simulink model "fullVehicleModel_17b"  (R2017b)
settings: Solver=VariableStepAuto  StartTime=0.0  StopTime=10.0  RelTol=1e-3
undefined symbols (not defined in the file): ambient_temp, bat, bat_r1, Batt, batt_initCharge, Batt_sensorLag_s, bvatt_AhRating, DiscIntNeverNeededParam, electronics_power, env, module_broad_area, module_small_area, module_top_area, mot, no_module, shifterPos, Ts, Ts_elec
libraries: Soft_ECUs x90, fl_lib x67, nesl_utility x29, Battery_lib x28, Gen_lib x13, simulink x10, aerolibconvert2 x7, SoftCAN_Interface x6, autolibshared x2, Additional_blocks_lib x1, elec_lib x1
(part 1 of 4)
settings Model: Creator=carca  LastModifiedBy=Truman

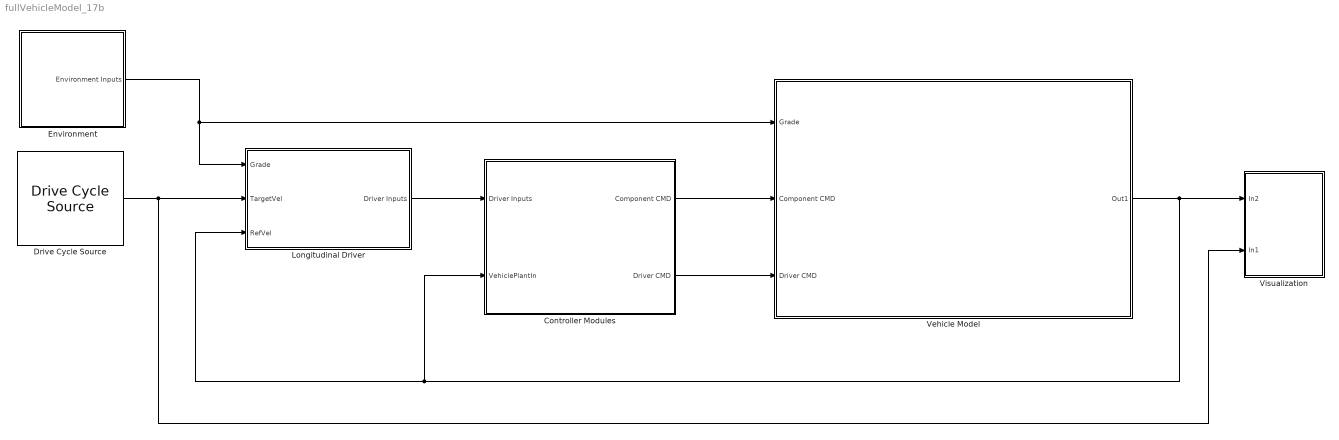
== system fullVehicleModel_17b ==
  "Controller Modules " : Subsystem
      mask Display: image('C:\Users\carca\Desktop\Icon Images\controllerMask.png');
  Drive Cycle Source : autolibshared/Drive Cycle Source  cycleVar=FTP75  fileVar=cycleFTP75.mat  tfinal="2474  seconds"  cycleRepeat=off  outAccPort=off  t_wot1=5  xdot_woto=0  xdot_wot1=30  t_wot2=20  xdot_wot2=0  t_wotend=30  srcUnit=m/s  outUnit=m/s  srcAccUnit=m/s/s  outAccUnit=m/s^2  dt=0
      settings: SourceProductName=Powertrain Blockset  SourceProductBaseCode=PW
  Environment : Subsystem
      mask Display: image('C:\Users\carca\Desktop\Icon Images\environmentMask.png');
  Longitudinal Driver : Subsystem
      mask Display: image('C:\Users\carca\Desktop\Icon Images\driverMask.png');
  Vehicle Model : Subsystem
      mask Display: image('C:\Users\carca\Desktop\Icon Images\camaroMask.png');
  "Visualization " : Subsystem
  wires:
  Environment/1(Environment Inputs) -> Longitudinal Driver/1(Grade), Vehicle Model/1(Grade)
  "Controller Modules "/1(Component CMD) -> Vehicle Model/2(Component CMD)
  "Controller Modules "/2("Driver CMD ") -> Vehicle Model/3(Driver CMD)
  Longitudinal Driver/1(Driver Inputs) -> "Controller Modules "/1(Driver Inputs)
  Vehicle Model/1(Out1) -> Longitudinal Driver/3(RefVel), "Controller Modules "/2(VehiclePlantIn), "Visualization "/1(In2)
  Drive Cycle Source/1 -> "Visualization "/2(In1), Longitudinal Driver/2(TargetVel)

== system fullVehicleModel_17b/Controller Modules  ==
  Driver Inputs : Inport
  VehiclePlantIn : Inport  Port=2
  Component Controllers : Subsystem
  Controller : Subsystem  Variant=on
  Controller Inputs : Subsystem  Variant=on
  Controller Outputs : Subsystem  Variant=on
  Component CMD : Outport
  "Driver CMD " : Outport  Port=2
  wires:
  Controller Inputs/1(ControllerInputs) -> Controller/1(In1)
  Controller/1(Out1) -> Controller Outputs/1(In1)
  Controller Outputs/1(Out1) -> Component Controllers/3(HSCSignals)
  Driver Inputs/1 -> Component Controllers/2(DriverInputs), "Driver CMD "/1, Controller Inputs/1(DriverInputs)
  VehiclePlantIn/1 -> Component Controllers/1(PlantSignals)
  Component Controllers/1(ToVehiclePlant) -> Component CMD/1
  Component Controllers/2(ToHSC) -> Controller Inputs/2(SystemInputs)

== system fullVehicleModel_17b/Environment ==
  Grade Input : FromWorkspace  VariableName=driveCycle.grade_deg  SampleTime=0
  Environment Inputs : Outport
  wires:
  Grade Input/1 -> Environment Inputs/1

== system fullVehicleModel_17b/Longitudinal Driver ==
  Grade : Inport
  TargetVel : Inport  Port=2
  RefVel : Inport  Port=3
  Driver Model : Subsystem
  Signal Process : Subsystem
  Driver Inputs : Outport
  wires:
  TargetVel/1 -> Driver Model/1(TargetVel)
  RefVel/1 -> Driver Model/2(VelFedbk)
  Driver Model/1(Driver_Inputs) -> Signal Process/1(Driver_Inputs)
  Signal Process/1(Driver_Signals) -> Driver Inputs/1
  Grade/1 -> Driver Model/3("Grade ")

== system fullVehicleModel_17b/Vehicle Model ==
  Grade : Inport
  Component CMD : Inport  Port=2
  Driver CMD : Inport  Port=3
  "Cooling System " : Subsystem
  "Drivetrain Model " : Subsystem
  Genset Plant : Subsystem
  Motor Plant : Subsystem
  Subsystem : Subsystem
  Variant Subsystem : Subsystem  Variant=on  OverrideUsingVariant=Variant
  Variant Subsystem1 : Subsystem  Variant=on  OverrideUsingVariant=Variant
  Variant Subsystem2 : Subsystem  Variant=on
  Out1 : Outport
  wires:
  Genset Plant/1(Out1) -> Variant Subsystem1/2(Genset Inputs)
  [ComponentCMD] -> Genset Plant/1(In1)
  [ComponentCMD] -> Variant Subsystem1/1(Component Cmds)
  [ComponentCMD] -> Variant Subsystem/1("Batt Commands ")
  [ComponentCMD] -> Motor Plant/1(In1)
  [DriverCMD] -> Variant Subsystem1/3(Driver Signals)
  [ComponentCMD] -> "Cooling System "/1(In1)
  [DriverCMD] -> "Cooling System "/2(In2)
  Variant Subsystem/1(Batt Signals) -> Subsystem/1(In1)
  ? -> Subsystem/2(In2)
  Motor Plant/1(Out1) -> Subsystem/3(In3)
  "Drivetrain Model "/1(Out1) -> Subsystem/4(In4)
  Component CMD/1 -> [ComponentCMD]
  Driver CMD/1 -> [DriverCMD]
  [ComponentCMD] -> Subsystem/5(In5)
  Subsystem/1(Out1) -> Out1/1
  Grade/1 -> [Grade]
  [Grade] -> "Drivetrain Model "/1(In1)
  connections:
  Variant Subsystem1/LConn1 -- Variant Subsystem/LConn1
  Variant Subsystem1/LConn2 -- Variant Subsystem/LConn2

== system fullVehicleModel_17b/Visualization  ==
  In2 : Inport
  In1 : Inport  Port=2

== system fullVehicleModel_17b/Controller Modules /Component Controllers ==
  PlantSignals : Inport
  DriverInputs : Inport  Port=2
  HSCSignals : Inport  Port=3
  BMS Control Module : Subsystem
  Bus Creator2 : BusCreator  Inputs=5
  Bus Creator3 : BusCreator  Inputs=5
  Bus Selector5 : BusSelector  OutputSignals=driver_inputs.drv_keyPos
  Genset Control Module : Subsystem
  INVCON Controller Module : Subsystem
  Left Motor Control Module : Subsystem
  Right Motor Control Module : Subsystem
  ToVehiclePlant : Outport
  ToHSC : Outport  Port=2
  wires:
  PlantSignals/1 -> Genset Control Module/2(VehPlant), INVCON Controller Module/2(INVPlantIn), Left Motor Control Module/2(MotorPlantSig), Right Motor Control Module/2(MotorPlantSig), BMS Control Module/2(BattPlantIn)
  HSCSignals/1 -> Genset Control Module/1(HSCGenIN), INVCON Controller Module/1(INVHSCIn), BMS Control Module/1(BattHSCIn), Left Motor Control Module/1(HSCInputs), Right Motor Control Module/1(HSCInputs)
  Bus Selector5/1 -> Left Motor Control Module/3(IgnitionCMD), Right Motor Control Module/3(IgnitionCMD), BMS Control Module/3(IgnitionCMD)  "<drv_keyPos>"
  Right Motor Control Module/1(Right_Motor_HSC) -> Bus Creator2/1
  Left Motor Control Module/1(Left_Motor_HSC) -> Bus Creator2/2
  BMS Control Module/1(BattToHSC) -> Bus Creator2/3
  INVCON Controller Module/1(INV_HSC) -> Bus Creator2/4
  Genset Control Module/1(GenSet_HSC) -> Bus Creator2/5
  Right Motor Control Module/2(Right_Motor_Plant) -> Bus Creator3/1
  Left Motor Control Module/2(Left_Motor_Plant) -> Bus Creator3/2
  BMS Control Module/2(Batt_plant) -> Bus Creator3/3
  INVCON Controller Module/2(INV_Plant) -> Bus Creator3/4
  Genset Control Module/2(GenSet_Plant) -> Bus Creator3/5
  DriverInputs/1 -> Bus Selector5/1
  Bus Creator2/1 -> ToHSC/1
  Bus Creator3/1 -> ToVehiclePlant/1

== system fullVehicleModel_17b/Controller Modules /Controller ==
  note: 1) Add Subsystem or Model blocks as valid variant choices.
      | 2) You cannot connect blocks at this level. At simulation, connectivity is automatically
      | determined, based on the active variant and port name matching.
  In1 : Inport
  HiL HSC Controller : Subsystem  VariantControl=Variant1
  SiL HSC Controller : Subsystem  VariantControl=Variant
  Out1 : Outport

== system fullVehicleModel_17b/Controller Modules /Controller Inputs ==
  note: 1) Add Subsystem or Model blocks as valid variant choices.
      | 2) You cannot connect blocks at this level. At simulation, connectivity is automatically
      | determined, based on the active variant and port name matching.
  DriverInputs : Inport
  SystemInputs : Inport  Port=2
  HiL Inputs : Subsystem  VariantControl=Variant1
  SiL Inputs : Subsystem  VariantControl=Variant
  ControllerInputs : Outport

== system fullVehicleModel_17b/Controller Modules /Controller Outputs ==
  note: 1) Add Subsystem or Model blocks as valid variant choices.
      | 2) You cannot connect blocks at this level. At simulation, connectivity is automatically
      | determined, based on the active variant and port name matching.
  In1 : Inport
  HiL Controller Outputs : Subsystem  VariantControl=Variant1
  SiL Controller Outputs : Subsystem  VariantControl=Variant
  Out1 : Outport

== system fullVehicleModel_17b/Longitudinal Driver/Driver Model ==
  TargetVel : Inport
  VelFedbk : Inport  Port=2
  "Grade " : Inport  Port=3
  Bus Creator : BusCreator  Inputs=5
  Driver Model : Subsystem  Variant=on
  Gear and Key Position : Subsystem
  Ground : Ground
  Pedal Procedure : Subsystem
  Vehicle Mode Selection : Subsystem
  Driver_Inputs : Outport
  wires:
  Driver Model/1(AccelCmd) -> Pedal Procedure/1(AccelCmd)
  Driver Model/2(BrkCmd) -> Pedal Procedure/2(BrkCmd)
  Bus Creator/1 -> Driver_Inputs/1  "Driver_Inputs"
  Gear and Key Position/1(KeyPos) -> Bus Creator/3  "drv_KeyPos"
  TargetVel/1 -> Driver Model/1(CmdVel)
  Pedal Procedure/2(BrklPos) -> Bus Creator/2  "drv_AccelPos_Percent"
  VelFedbk/1 -> Driver Model/3(VelFdbk), Gear and Key Position/1(VehSpd)
  Gear and Key Position/2(GearPos) -> Pedal Procedure/3(GearPos), Bus Creator/4  "drv_GearPos"
  Pedal Procedure/1(AccelPos) -> Bus Creator/1  "drv_BrkPos_Percent"
  Vehicle Mode Selection/1(VehModeCmd) -> Bus Creator/5  "drv_VehModeCmd"
  Ground/1 -> Vehicle Mode Selection/1(VehModeRequest)
  "Grade "/1 -> Driver Model/2("Grade ")

== system fullVehicleModel_17b/Longitudinal Driver/Signal Process ==
  Driver_Inputs : Inport
  Bus Creator : BusCreator  Inputs=12
  Bus Selector : BusSelector  OutputSignals=drv_AccelPos_Percent,drv_BrkPos_Percent,drv_KeyPos,drv_GearPos,drv_PerfModeReq,drv_RegenDisableReq,drv_FuelConvReq,drv_CsModeReq
  Constant : Constant
  acc_pwr_status : Constant
  Driver_Signals : Outport
  wires:
  Driver_Inputs/1 -> Bus Selector/1
  Bus Selector/2 -> Bus Creator/3, Bus Creator/2  "<drv_BrkPos_Percent>"
  Bus Selector/1 -> Bus Creator/1  "<drv_AccelPos_Percent>"
  Bus Selector/3 -> Bus Creator/4  "<drv_KeyPos>"
  Bus Selector/4 -> Bus Creator/5  "<drv_GearPos>"
  Bus Selector/5 -> Bus Creator/6  "<drv_PerfModeReq>"
  Bus Selector/6 -> Bus Creator/7  "<drv_RegenDisableReq>"
  Bus Selector/7 -> Bus Creator/8  "<drv_FuelConvReq>"
  Bus Selector/8 -> Bus Creator/9  "<drv_CsModeReq>"
  acc_pwr_status/1 -> Bus Creator/10
  Constant/1 -> Bus Creator/11, Bus Creator/12
  Bus Creator/1 -> Driver_Signals/1

== system fullVehicleModel_17b/Vehicle Model/Cooling System  ==
  In1 : Inport
  In2 : Inport  Port=2

== system fullVehicleModel_17b/Vehicle Model/Drivetrain Model  ==
  In1 : Inport
  Out1 : Outport
  wires:
  In1/1 -> Out1/1

== system fullVehicleModel_17b/Vehicle Model/Genset Plant ==
  In1 : Inport
  GenSet Plant : Subsystem
  GenSet Plant Input : Subsystem
  Subsystem : Subsystem
  Out1 : Outport
  wires:
  GenSet Plant Input/1(Out1) -> GenSet Plant/1(EngineThrottleReq)
  GenSet Plant Input/3(Out3) -> GenSet Plant/3(EnableSignal)
  GenSet Plant Input/2(Out2) -> GenSet Plant/2(GenLoadTrqReq)
  In1/1 -> GenSet Plant Input/1(In1)
  GenSet Plant/1(Out1) -> Subsystem/1(In1)
  GenSet Plant/2(Out2) -> Subsystem/2(In2)
  GenSet Plant/3(Out3) -> Subsystem/3(In3)
  GenSet Plant/4(Out4) -> Subsystem/4(In4)
  GenSet Plant/5(Out5) -> Subsystem/5(In5)
  GenSet Plant/6(Out6) -> Subsystem/6(In6)
  GenSet Plant/7(Out7) -> Subsystem/7(In7)
  GenSet Plant/8(Out8) -> Subsystem/8(In8)
  GenSet Plant/9(Out9) -> Subsystem/9(In9)
  GenSet Plant/10(Out10) -> Subsystem/10(In10)
  GenSet Plant/11(Out11) -> Subsystem/11(In11)
  Subsystem/1(Out1) -> Out1/1

== system fullVehicleModel_17b/Vehicle Model/Motor Plant ==
  In1 : Inport
  Out1 : Outport
  wires:
  In1/1 -> Out1/1

== system fullVehicleModel_17b/Vehicle Model/Subsystem ==
  In1 : Inport
  In2 : Inport  Port=2
  In3 : Inport  Port=3
  In4 : Inport  Port=4
  In5 : Inport  Port=5
  Bus Creator : BusCreator  Inputs=5
  Out1 : Outport
  wires:
  In1/1 -> Bus Creator/1
  In2/1 -> Bus Creator/2
  In3/1 -> Bus Creator/3
  Bus Creator/1 -> Out1/1
  In4/1 -> Bus Creator/4
  In5/1 -> Bus Creator/5

== system fullVehicleModel_17b/Vehicle Model/Variant Subsystem ==
  note: 1) Add Subsystem or Model blocks as valid variant choices.
      | 2) You cannot connect blocks at this level. At simulation, connectivity is automatically
      | determined, based on the active variant and port name matching.
  "Batt Commands " : Inport
  Subsystem : Subsystem  VariantControl=Variant
  Subsystem1 : Subsystem  VariantControl=Variant1
  Subsystem2 : Subsystem  VariantControl=Variant2
  Batt_+ : PMIOPort  Port=1  Side=Left
  Batt_- : PMIOPort  Port=2  Side=Left
  Batt Signals : Outport

== system fullVehicleModel_17b/Vehicle Model/Variant Subsystem1 ==
  note: 1) Add Subsystem or Model blocks as valid variant choices.
      | 2) You cannot connect blocks at this level. At simulation, connectivity is automatically
      | determined, based on the active variant and port name matching.
  Component Cmds : Inport
  Genset Inputs : Inport  Port=2
  Driver Signals : Inport  Port=3
  Subsystem : Subsystem  VariantControl=Variant
  Subsystem1 : Subsystem  VariantControl=Variant1
  Batt_+ : PMIOPort  Port=1  Side=Left
  " Batt_-" : PMIOPort  Port=2  Side=Left
  Out1 : Outport

== system fullVehicleModel_17b/Vehicle Model/Variant Subsystem2 ==
  note: 1) Add Subsystem or Model blocks as valid variant choices.
      | 2) You cannot connect blocks at this level. At simulation, connectivity is automatically
      | determined, based on the active variant and port name matching.
  In1 : Inport
  Subsystem : Subsystem  VariantControl=Variant
  Subsystem1 : Subsystem  VariantControl=Variant1
  Out1 : Outport

== system fullVehicleModel_17b/Controller Modules /Component Controllers/BMS Control Module ==
  BattHSCIn : Inport
  BattPlantIn : Inport  Port=2
  IgnitionCMD : Inport  Port=3
  BMS Controller Module : Subsystem
  Controller Inputs : Subsystem  Variant=on
  Controller Outputs : Subsystem  Variant=on
  BattToHSC : Outport
  Batt_plant : Outport  Port=2
  wires:
  BattHSCIn/1 -> Controller Inputs/1(BattHSC)
  Controller Inputs/1(BMS_BMSEnable) -> BMS Controller Module/1(BMS_BMSEnable)
  BMS Controller Module/1(Out1) -> Controller Outputs/1(In1)
  Controller Outputs/1(Out1) -> Batt_plant/1
  Controller Inputs/2(BMS_BMSEPO) -> BMS Controller Module/2(BMS_BMSEPO)
  Controller Inputs/3(BMS_mainContctClose) -> BMS Controller Module/3(BMS_mainContctClose)
  Controller Inputs/4(Batt_current_A) -> BMS Controller Module/4(Batt_current_A)
  Controller Inputs/5(Batt_SOC_pct) -> BMS Controller Module/5(Batt_SOC_pct)
  Controller Inputs/6(Batt_temp_C) -> BMS Controller Module/6(Batt_temp_C)
  Controller Inputs/7(Batt_voltage_V) -> BMS Controller Module/7(Batt_voltage_V)
  Controller Inputs/8(IngnitionCMD) -> BMS Controller Module/8(IgnitionCMD)
  BMS Controller Module/2(Out2) -> Controller Outputs/2(In2)
  Controller Outputs/2(Out2) -> BattToHSC/1
  BattPlantIn/1 -> Controller Inputs/2(BattPlant)
  IgnitionCMD/1 -> Controller Inputs/3(IgnitionCMD)

== system fullVehicleModel_17b/Controller Modules /Component Controllers/Genset Control Module ==
  HSCGenIN : Inport
  VehPlant : Inport  Port=2
  Controller Inputs : Subsystem  Variant=on
  Controller Outputs : Subsystem  Variant=on
  Genset Controller Module : Subsystem
  GenSet_HSC : Outport
  GenSet_Plant : Outport  Port=2
  wires:
  HSCGenIN/1 -> Controller Inputs/1(HSCCmd)
  Controller Inputs/1(eng_starterSwitchReq_bool) -> Genset Controller Module/1(In1)
  Genset Controller Module/1(Out1) -> Controller Outputs/1(eng_enable)
  Controller Outputs/1(ToHSC) -> GenSet_HSC/1
  Controller Inputs/2(Out2) -> Genset Controller Module/2(In2)
  Controller Inputs/3(Out3) -> Genset Controller Module/3(In3)
  Controller Inputs/4(Out4) -> Genset Controller Module/4(In4)
  Controller Inputs/5(Out5) -> Genset Controller Module/5(In5)
  Controller Inputs/6(Out6) -> Genset Controller Module/6(In6)
  Controller Inputs/7(Out7) -> Genset Controller Module/7(In7)
  Genset Controller Module/2(Out2) -> Controller Outputs/2(eng_throttleReq_pct)
  Genset Controller Module/3(Out3) -> Controller Outputs/3(gen_enable)
  Genset Controller Module/4(Out4) -> Controller Outputs/4(gen_loadTrqReq_Nm)
  Genset Controller Module/5(Out5) -> Controller Outputs/5(gen_pwrElec_kW)
  Genset Controller Module/6(Out6) -> Controller Outputs/6(eng_engineSpd_rpm)
  Genset Controller Module/7(Out7) -> Controller Outputs/7(eng_fuelLevelBit_bool)
  Controller Outputs/2(PlantCmds) -> GenSet_Plant/1
  VehPlant/1 -> Controller Inputs/2(VehPlant)
  Controller Inputs/8(Out8) -> Genset Controller Module/8(gen_pwrElec_kW)
  Controller Inputs/10(Out10) -> Genset Controller Module/10(eng_fuelLevelBit_bool)
  Controller Inputs/9(Out9) -> Genset Controller Module/9(eng_engineSpd_rpm)

== system fullVehicleModel_17b/Controller Modules /Component Controllers/INVCON Controller Module ==
  INVHSCIn : Inport
  INVPlantIn : Inport  Port=2
  Controller Inputs : Subsystem  Variant=on  OverrideUsingVariant=Variant
  Controller Outputs : Subsystem  Variant=on  OverrideUsingVariant=Variant
  INVCON Controller Module : Subsystem
  INV_HSC : Outport
  INV_Plant : Outport  Port=2
  wires:
  INVHSCIn/1 -> Controller Inputs/1(HSCCmd)
  INVCON Controller Module/1(HV_DCVoltage_V) -> Controller Outputs/1(HV_DCVoltage_V)
  Controller Inputs/1(HV_Dmd) -> INVCON Controller Module/1(HV_Dmd)
  Controller Inputs/2(HV_CurrDmd) -> INVCON Controller Module/2(HV_CurrDmd)
  Controller Inputs/3(LV_CurrDmd) -> INVCON Controller Module/3(LV_CurrDmd)
  Controller Inputs/4(LV_Dmd) -> INVCON Controller Module/4(LV_Dmd)
  Controller Inputs/5(DCDC_ModeReq) -> INVCON Controller Module/5(DCDC_ModeReq)
  Controller Inputs/6(HV_current) -> INVCON Controller Module/6(HV_current_A)
  Controller Inputs/7(HV_volt) -> INVCON Controller Module/7(HV_Voltage_V)
  Controller Inputs/8(Aux_load) -> INVCON Controller Module/8(Aux_load)
  Controller Inputs/9(gen_GenCurrent_A) -> INVCON Controller Module/9(gen_GenCurrent_A)
  Controller Inputs/10(gen_loadTrq_Nm) -> INVCON Controller Module/10(gen_loadTrq_Nm)
  INVCON Controller Module/2(LV_DCCurrent_A) -> Controller Outputs/2(LV_DCCurrent_A)
  INVCON Controller Module/3(DC_Mode) -> Controller Outputs/3(DC_Mode)
  INVCON Controller Module/4(HV_DCCurrent_A) -> Controller Outputs/4(HV_DCCurrent_A)
  INVCON Controller Module/5(DC_Temp) -> Controller Outputs/5(DC_Temp)
  INVCON Controller Module/6(LV_DCVoltage_V) -> Controller Outputs/6(LV_DCVoltage_V)
  INVCON Controller Module/7(gen_GenCurrent_A1) -> Controller Outputs/7(gen_GenCurrent_A)
  INVCON Controller Module/8(gen_loadTrq_Nm1) -> Controller Outputs/8(gen_loadTrq_Nm)
  INVPlantIn/1 -> Controller Inputs/2(VehPlant)
  Controller Outputs/1(INVToHSC) -> INV_Plant/1, INV_HSC/1

== system fullVehicleModel_17b/Controller Modules /Component Controllers/Left Motor Control Module ==
  HSCInputs : Inport
  MotorPlantSig : Inport  Port=2
  IgnitionCMD : Inport  Port=3
  Controller : Subsystem
  Controller Inputs : Subsystem  Variant=on
  Controller Outputs : Subsystem  Variant=on
  Left_Motor_HSC : Outport
  Left_Motor_Plant : Outport  Port=2
  wires:
  HSCInputs/1 -> Controller Inputs/1(HSC Inputs)
  Controller Outputs/1(MotorToHSC) -> Left_Motor_HSC/1
  Controller/1(fualtDiag) -> Controller Outputs/1(FaultDiagnos)
  Controller/2(Mot_Signals) -> Controller Outputs/2(MotorSignals)
  Controller/3(startupSignals) -> Controller Outputs/3(StartupSignals)
  Controller/4(motorState) -> Controller Outputs/4(MotorState)
  Controller/5(Motor_CMD) -> Controller Outputs/5(MotorCMD)
  Controller/6(StatusReqREGID) -> Controller Outputs/6(StatusRequest)
  Controller Outputs/2(MotorTrqCMD) -> Left_Motor_Plant/1
  MotorPlantSig/1 -> Controller Inputs/2(Motor Signals)
  IgnitionCMD/1 -> Controller Inputs/3(Ignition)
  Controller Inputs/1(mot_trqCmd_pct) -> Controller/1(mot_trqCmd_pct)
  Controller Inputs/2(mot_pwrMech_kW) -> Controller/2(mot_pwrMech_kW)
  Controller Inputs/3(mot_motSpd_RPM) -> Controller/3(mot_motSpd_RPM)
  Controller Inputs/4(mot_pwrElec_kW) -> Controller/4(mot_pwrElec_kW)
  Controller Inputs/5(mot_motEff_k) -> Controller/5(mot_motEff_k)
  Controller Inputs/6(mot_temp) -> Controller/6(mot_temp)
  Controller Inputs/7(mot_current) -> Controller/7(mot_current)
  Controller Inputs/8(mot_voltage) -> Controller/8(mot_voltage)
  Controller Inputs/9(mot_currentSensor) -> Controller/9(mot_currentSensor)
  Controller Inputs/10(mot_modeEnable) -> Controller/10(mot_modeEnable)
  Controller Inputs/11(Info) -> Controller/11(info)
  Controller Inputs/12(Ignition1) -> Controller/12(ignition)

== system fullVehicleModel_17b/Controller Modules /Component Controllers/Right Motor Control Module ==
  HSCInputs : Inport
  MotorPlantSig : Inport  Port=2
  IgnitionCMD : Inport  Port=3
  Controller Inputs : Subsystem  Variant=on
  Controller Outputs : Subsystem  Variant=on
  Subsystem : Subsystem
  Right_Motor_HSC : Outport
  Right_Motor_Plant : Outport  Port=2
  wires:
  HSCInputs/1 -> Controller Inputs/1(In1)
  Controller Outputs/1(MotorToHSC) -> Right_Motor_HSC/1
  Controller Inputs/1(Out1) -> Subsystem/1(In1)
  Subsystem/1(Out1) -> Controller Outputs/1(FaultDiagnos)
  Controller Inputs/2(Out2) -> Subsystem/2(In2)
  Controller Inputs/3(Out3) -> Subsystem/3(In3)
  Controller Inputs/4(Out4) -> Subsystem/4(In4)
  Controller Inputs/5(Out5) -> Subsystem/5(In5)
  Controller Inputs/6(Out6) -> Subsystem/6(In6)
  Controller Inputs/7(Out7) -> Subsystem/7(In7)
  Controller Inputs/8(Out8) -> Subsystem/8(In8)
  Controller Inputs/9(Out9) -> Subsystem/9(In9)
  Controller Inputs/10(Out10) -> Subsystem/10(In10)
  Controller Inputs/11(Out11) -> Subsystem/11(In11)
  Controller Inputs/12(Out12) -> Subsystem/12(In12)
  Subsystem/2(Out2) -> Controller Outputs/2(MotorSignals)
  Subsystem/3(Out3) -> Controller Outputs/3(StartupSignals)
  Subsystem/4(Out4) -> Controller Outputs/4(MotorState)
  Subsystem/5(Out5) -> Controller Outputs/5(MotorCMD)
  Subsystem/6(Out6) -> Controller Outputs/6(StatusRequest)
  Controller Outputs/2(MotorTrqCMD) -> Right_Motor_Plant/1
  MotorPlantSig/1 -> Controller Inputs/2(In2)
  IgnitionCMD/1 -> Controller Inputs/3(In3)

== system fullVehicleModel_17b/Controller Modules /Controller/HiL HSC Controller ==
  In1 : Inport
  Out1 : Outport

== system fullVehicleModel_17b/Controller Modules /Controller/SiL HSC Controller ==
  In1 : Inport
  Out1 : Outport

== system fullVehicleModel_17b/Controller Modules /Controller Inputs/HiL Inputs ==
  DriverInputs : Inport
  ControllerInputs : Outport

== system fullVehicleModel_17b/Controller Modules /Controller Inputs/SiL Inputs ==
  DriverInputs : Inport
  SystemInputs : Inport  Port=2
  Bus Creator : BusCreator  Inputs=6
  Bus Creator1 : BusCreator  Inputs=2
  Bus Selector3 : BusSelector  OutputSignals=mot_R_SoftCAN_Outputs,BMS_SoftCAN_Outputs,mot_L_SoftCAN_Outputs,driver_sigs,INVCON_SoftCAN_Outputs,genset_softECU_toHSC
  Rename : SoftCAN_Interface/HSC_In/Rename
  Rename1 : SoftCAN_Interface/HSC_In/Rename1
  Rename2 : SoftCAN_Interface/HSC_In/Rename2
  Rename3 : SoftCAN_Interface/HSC_In/Rename3
  Rename4 : SoftCAN_Interface/HSC_In/Rename4
  Signal Mapping : SoftCAN_Interface/HSC_In/Signal Mapping
  ControllerInputs : Outport
  wires:
  Rename2/1 -> Bus Creator/6  "genset_signal_out"
  Bus Selector3/4 -> Rename1/1  "<driver_sigs>"
  Bus Creator/1 -> ControllerInputs/1
  Bus Selector3/2 -> Rename/1  "<BMS_SoftCAN_Outputs>"
  Rename/1 -> Bus Creator/2  "ess_signal_out"
  Bus Selector3/6 -> Rename2/1  "<genset_softECU_toHSC>"
  Rename3/1 -> Bus Creator/1  "rtmRight_signal_out"
  Bus Selector3/1 -> Rename3/1  "<mot_R_SoftCAN_Outputs>"
  Bus Selector3/5 -> Signal Mapping/1  "<INVCON_SoftCAN_Outputs>"
  Rename4/1 -> Bus Creator/3  "rtmLeft_signal_out"
  Bus Selector3/3 -> Rename4/1  "<mot_L_SoftCAN_Outputs>"
  Rename1/1 -> Bus Creator/4  "driver_signal_out"
  Signal Mapping/1 -> Bus Creator/5  "invcon_signal_out"
  SystemInputs/1 -> Bus Creator1/2
  DriverInputs/1 -> Bus Creator1/1
  Bus Creator1/1 -> Bus Selector3/1

== system fullVehicleModel_17b/Controller Modules /Controller Outputs/HiL Controller Outputs ==
  In1 : Inport
  Out1 : Outport

== system fullVehicleModel_17b/Controller Modules /Controller Outputs/SiL Controller Outputs ==
  In1 : Inport
  Out1 : Outport

== system fullVehicleModel_17b/Longitudinal Driver/Driver Model/Driver Model ==
  note: 1) Add Subsystem or Model blocks as valid variant choices.
      | 2) You cannot connect blocks at this level. At simulation, connectivity is automatically
      | determined, based on the active variant and port name matching.
  CmdVel : Inport
  "Grade " : Inport  Port=2
  VelFdbk : Inport  Port=3
  Classic Driver : Subsystem  VariantControl=Variant1
  Thermostatic Driver : Subsystem  VariantControl=Variant
  AccelCmd : Outport
  BrkCmd : Outport  Port=2

== system fullVehicleModel_17b/Longitudinal Driver/Driver Model/Gear and Key Position ==
  VehSpd : Inport
  KeyPos : Outport
  GearPos : Outport  Port=2

== system fullVehicleModel_17b/Longitudinal Driver/Driver Model/Pedal Procedure ==
  note: script value
  note: No acceleration if brake is more than 0.5%
  note: if shifter not in Drive, 100% brake
  AccelCmd : Inport
  BrkCmd : Inport  Port=2
  GearPos : Inport  Port=3
  Compare To Constant : simulink/Logic and Bit Operations/Compare To Constant  relop===  const=shifterPos.drive  OutDataTypeStr=boolean
  Constant : Constant  Value=0
  Constant1 : Constant  Value=0
  Constant2 : Constant  Value=100
  Gain : Gain  Gain=100
  Gain1 : Gain  Gain=100
  Switch : Switch  Criteria=u2 > Threshold
  Switch1 : Switch  Criteria=u2 > Threshold
  Switch2 : Switch  Criteria=u2 > Threshold  Threshold=0.5
  AccelPos : Outport
  BrklPos : Outport  Port=2
  wires:
  Switch/1 -> BrklPos/1  "drv_brakePos_Percent"
  Compare To Constant/1 -> Switch1/2, Switch/2
  GearPos/1 -> Compare To Constant/1
  Constant1/1 -> Switch2/1
  Constant2/1 -> Switch/3
  Gain1/1 -> Switch2/2, Switch/1  "drv_brakePos_Percent"
  Gain/1 -> Switch1/1  "drv_accelPos_Percent"
  AccelCmd/1 -> Gain/1
  Switch2/1 -> AccelPos/1  "drv_accelPos_Percent"
  BrkCmd/1 -> Gain1/1
  Switch1/1 -> Switch2/3  "drv_accelPos_Percent"
  Constant/1 -> Switch1/3

== system fullVehicleModel_17b/Longitudinal Driver/Driver Model/Vehicle Mode Selection ==
  VehModeRequest : Inport
  Bus Creator1 : BusCreator  Inputs=4
  Terminator : Terminator
  drv_CsModeReq : Constant  Value=0
  drv_FuelConvReq : Constant  Value=0
  drv_PerfModeReq : Constant  Value=0
  drv_RegenDisableReq : Constant  Value=0
  VehModeCmd : Outport
  wires:
  drv_FuelConvReq/1 -> Bus Creator1/3  "drv_FuelConvReq"
  drv_PerfModeReq/1 -> Bus Creator1/1  "drv_PerfModeReq"
  drv_RegenDisableReq/1 -> Bus Creator1/2  "drv_RegenDisableReq"
  drv_CsModeReq/1 -> Bus Creator1/4  "drv_CsModeReq"
  Bus Creator1/1 -> VehModeCmd/1
  VehModeRequest/1 -> Terminator/1

== system fullVehicleModel_17b/Vehicle Model/Genset Plant/GenSet Plant ==
  EngineThrottleReq : Inport
  GenLoadTrqReq : Inport  Port=2
  EnableSignal : Inport  Port=3
  Out1 : Outport
  Out2 : Outport  Port=2
  Out3 : Outport  Port=3
  Out4 : Outport  Port=4
  Out5 : Outport  Port=5
  Out6 : Outport  Port=6
  Out7 : Outport  Port=7
  Out8 : Outport  Port=8
  Out9 : Outport  Port=9
  Out10 : Outport  Port=10
  Out11 : Outport  Port=11
  wires:
  EngineThrottleReq/1 -> ?
  GenLoadTrqReq/1 -> ?
  EnableSignal/1 -> ?

== system fullVehicleModel_17b/Vehicle Model/Genset Plant/GenSet Plant Input ==
  In1 : Inport
  Bus Selector9 : BusSelector  OutputSignals=eng_throttleReq_pct,gen_loadTrqReq_Nm,enableSig
  Out1 : Outport
  Out2 : Outport  Port=2
  Out3 : Outport  Port=3
  wires:
  In1/1 -> Bus Selector9/1
  Bus Selector9/2 -> Out2/1  "<gen_loadTrqReq_Nm>"
  Bus Selector9/3 -> Out3/1  "<enableSig>"
  Bus Selector9/1 -> Out1/1  "<eng_throttleReq_pct>"

== system fullVehicleModel_17b/Vehicle Model/Genset Plant/Subsystem ==
  In1 : Inport
  In2 : Inport  Port=2
  In3 : Inport  Port=3
  In4 : Inport  Port=4
  In5 : Inport  Port=5
  In6 : Inport  Port=6
  In7 : Inport  Port=7
  In8 : Inport  Port=8
  In9 : Inport  Port=9
  In10 : Inport  Port=10
  In11 : Inport  Port=11
  Out1 : Outport
  wires:
  In1/1 -> Out1/1

== system fullVehicleModel_17b/Vehicle Model/Variant Subsystem/Subsystem ==
  note: Battery Thermal
  note: Battery Dynamics
  note: Battery Sensors
  note: Battery Contactors
  "Batt Commands " : Inport
  Batt Current Sensor : fl_lib/Electrical/Electrical Sensors/Current Sensor
  Batt Voltage Sensor : fl_lib/Electrical/Electrical Sensors/Voltage Sensor
  Battery Dynamics : Subsystem
  Battery Thermal : Subsystem
  Capacitor : elec_lib/Passive Devices/Capacitor  enable_table=0  c=1e-6 F  Cvec=[1e-05, 1e-06] F  Vvec=[0, 10] V  CV_table_symmetry=1  C_tol=5  enable_C_tol=0  tol_distribution=1  nSigma=4  r=1e-6 Ohm  g=0 1/Ohm  enable_operating_limits=0  operating_limit_action=2  max_working_voltage_range=[-25, 25] V  power_rating=1 W  enable_faults=0  fault_action=1  Cscale_faulted=100  R_faulted=1e-3 Ohm  G_faulted=0 1/Ohm  tau_fault=1e-3 s  enable_temporal_fault=0  t_fault=1 s  enable_behavioral_fault=0  max_permissible_voltage_range=[-100, 100] V  t_fail_on_voltage=1 s  i_specify=off  i_priority=None  i=0 A  i_nominal_specify=off  i_nominal_unit=A  i_nominal_value=1  v_specify=off  v_priority=None  v=0 V  v_nominal_specify=off  v_nominal_unit=V  v_nominal_value=1  vc_specify=off  vc_priority=High  vc=0 V  vc_nominal_specify=off  vc_nominal_unit=V  vc_nominal_value=1
  Controlled Voltage Source1 : fl_lib/Electrical/Electrical Sources/Controlled Voltage Source
  Data Type Conversion : DataTypeConversion  OutDataTypeStr=double
  Electrical Reference1 : fl_lib/Electrical/Electrical Elements/Electrical Reference
  Input Signal Process : Subsystem
  Logical Operator1 : Logic  Operator=NOT  AllPortsSameDT=off  OutDataTypeStr=boolean
  Output Signal Processing : Subsystem
  Resistor : fl_lib/Electrical/Electrical Elements/Resistor  R=1 Ohm  i_specify=off  i_priority=None  i=0 A  i_nominal_specify=off  i_nominal_unit=A  i_nominal_value=1  v_specify=off  v_priority=None  v=0 V  v_nominal_specify=off  v_nominal_unit=V  v_nominal_value=1
  Simulink-PS Converter2 : nesl_utility/Simulink-PS Converter  PhysicalDomain=network_engine_domain  SubClassName=ps_input  LeftPortType=input  RightPortType=output  PseudoPeriodic=off  Frequencies=[]  NoiseDistribution=none  NoiseParameters=[]  Unit=1  AffineConversion=off  FilteringAndDerivatives=provide  SimscapeFilterOrder=1  InputFilterTimeConstant=0.001  UdotUserProvided=0
  Simulink-PS Converter3 : nesl_utility/Simulink-PS Converter  PhysicalDomain=network_engine_domain  SubClassName=ps_input  LeftPortType=input  RightPortType=output  PseudoPeriodic=off  Frequencies=[]  NoiseDistribution=none  NoiseParameters=[]  Unit=1  AffineConversion=off  FilteringAndDerivatives=provide  SimscapeFilterOrder=1  InputFilterTimeConstant=0.001  UdotUserProvided=0
  Solver Configuration : nesl_utility/Solver Configuration  PhysicalDomain=network_engine_domain  SubClassName=solver  LeftPortType=input  RightPortType=generic  Accelerate=off  Tones=[]  Harmonics=[]  SimulateNoise=off  Profile=off  UseLocalSampling=off  EnableSwitchedLinearOptims=on  FrequencyDomain=off  UseCCode=off  RelTol=0.001  AbsTol=1e-06  MinStep=1e-09  ToWorkspace=off  RevertToSquareIcSolve=off  NumHomotopyIterations=100  PhasorMode=off  PhasorModeNumHarmonics=1  DoDC=off  ResidualTolerance=1e-09  UseLocalSolver=off  LocalSolverChoice=NE_BACKWARD_EULER_ADVANCER  LocalSolverSampleTime=0.001  DoFixedCost=off  MaxNonlinIter=3  MaxModeIter=2  LinearAlgebra=Sparse  DelaysMemoryBudget=1024  AutomaticFiltering=on  FilteringTimeConstant=0.001
  Switch : fl_lib/Electrical/Electrical Elements/Switch  R_closed=0.01 Ohm  G_open=1e-8 1/Ohm  Threshold=0  i_specify=off  i_priority=None  i=0 A  i_nominal_specify=off  i_nominal_unit=A  i_nominal_value=1  v_specify=off  v_priority=None  v=0 V  v_nominal_specify=off  v_nominal_unit=V  v_nominal_value=1
      settings: SourceProductName=Simscape
  Switch1 : fl_lib/Electrical/Electrical Elements/Switch  R_closed=0.01 Ohm  G_open=1e-8 1/Ohm  Threshold=0  i_specify=off  i_priority=None  i=0 A  i_nominal_specify=off  i_nominal_unit=A  i_nominal_value=1  v_specify=off  v_priority=None  v=0 V  v_nominal_specify=off  v_nominal_unit=V  v_nominal_value=1
      settings: SourceProductName=Simscape
  Switch2 : fl_lib/Electrical/Electrical Elements/Switch  R_closed=0.01 Ohm  G_open=1e-8 1/Ohm  Threshold=0  i_specify=off  i_priority=None  i=0 A  i_nominal_specify=off  i_nominal_unit=A  i_nominal_value=1  v_specify=off  v_priority=None  v=0 V  v_nominal_specify=off  v_nominal_unit=V  v_nominal_value=1
      settings: SourceProductName=Simscape
  Batt_+ : PMIOPort  Port=1  Side=Left
  Batt_- : PMIOPort  Port=2  Side=Left
  Batt Signals : Outport
  wires:
  "Batt Commands "/1 -> Input Signal Process/1(In1)
  Input Signal Process/1(Contactor Cmd) -> Logical Operator1/1, Simulink-PS Converter2/1
  Logical Operator1/1 -> Data Type Conversion/1
  Data Type Conversion/1 -> Simulink-PS Converter3/1
  Battery Thermal/1(bat_temp) -> Output Signal Processing/1(Battery Temp)
  Output Signal Processing/1(Battery Measurements) -> Battery Dynamics/1(Batt Signals), Batt Signals/1
  connections:
  Capacitor/RConn1 -- Resistor/RConn1 -- Switch1/LConn1 -- Batt_-/RConn1
  Capacitor/LConn1 -- Switch2/LConn1 -- Switch/LConn1 -- Batt_+/RConn1
  Resistor/LConn1 -- Switch2/RConn2
  Simulink-PS Converter2/RConn1 -- Switch1/RConn1 -- Switch/RConn1
  Simulink-PS Converter3/RConn1 -- Switch2/RConn1
  Switch/RConn2 -- Batt Voltage Sensor/LConn1 -- Solver Configuration/RConn1 -- Controlled Voltage Source1/LConn1
  Switch1/RConn2 -- Batt Voltage Sensor/RConn2 -- Batt Current Sensor/RConn2
  Batt Current Sensor/LConn1 -- Electrical Reference1/LConn1 -- Controlled Voltage Source1/RConn2
  Controlled Voltage Source1/RConn1 -- Battery Dynamics/RConn1
  Batt Current Sensor/RConn1 -- Output Signal Processing/LConn2 -- Battery Thermal/LConn1
  Batt Voltage Sensor/RConn1 -- Output Signal Processing/LConn1

== system fullVehicleModel_17b/Vehicle Model/Variant Subsystem/Subsystem1 ==
  "Batt Commands " : Inport
  Batt_+ : PMIOPort  Port=1  Side=Left
  Batt_- : PMIOPort  Port=2  Side=Left
  Batt Signals : Outport

== system fullVehicleModel_17b/Vehicle Model/Variant Subsystem/Subsystem2 ==
  "Batt Commands " : Inport
  Batt_+ : PMIOPort  Port=1  Side=Left
  Batt_- : PMIOPort  Port=2  Side=Left
  Batt Signals : Outport

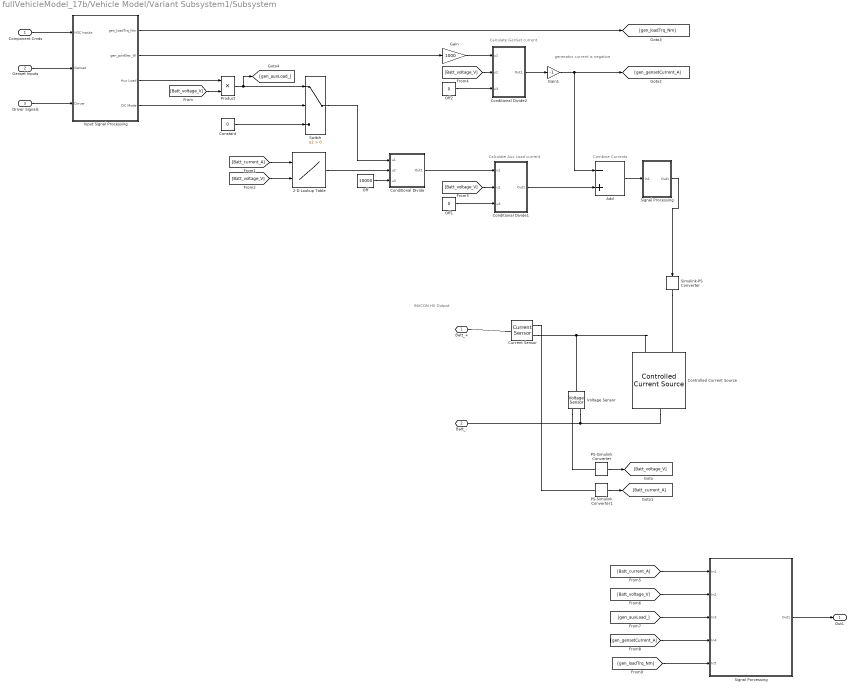
== system fullVehicleModel_17b/Vehicle Model/Variant Subsystem1/Subsystem ==
  note: generator current
      | is negative
  note: Combine Currents
  note: Calculate GenSet current
  note: Calculate Aux Load current
  note: INVCON HV Output
  Component Cmds : Inport
  Genset Inputs : Inport  Port=2
  Driver Signals : Inport  Port=3
  2-D Lookup Table : Lookup_n-D  BreakpointsForDimension1=[1:3]  BreakpointsForDimension2=[1:3]  InternalRulePriority=Speed  RndMeth=Simplest  InputSameDT=on
  Add : Sum  Inputs=-+
  Conditional Divide : Subsystem
  Conditional Divide1 : Subsystem
  Conditional Divide2 : Subsystem
  Constant : Constant  Value=0
  Controlled Current Source : fl_lib/Electrical/Electrical Sources/Controlled Current Source
  Current Sensor : fl_lib/Electrical/Electrical Sensors/Current Sensor
  Gain : Gain  Gain=1000
  Gain1 : Gain  Gain=-1
  Input Signal Processing : Subsystem  Variant=on
  Off : Constant  Value=10000
  Off1 : Constant  Value=0
  Off2 : Constant  Value=0
  PS-Simulink Converter : nesl_utility/PS-Simulink Converter  PhysicalDomain=network_engine_domain  SubClassName=ps_output  LeftPortType=input  RightPortType=output  PseudoPeriodic=off  Frequencies=[]  Unit=1  AffineConversion=off
  PS-Simulink Converter1 : nesl_utility/PS-Simulink Converter  PhysicalDomain=network_engine_domain  SubClassName=ps_output  LeftPortType=input  RightPortType=output  PseudoPeriodic=off  Frequencies=[]  Unit=1  AffineConversion=off
  Product : Product
  Signal Porcessing : Subsystem
  Signal Processing : Subsystem
  Simulink-PS Converter : nesl_utility/Simulink-PS Converter  PhysicalDomain=network_engine_domain  SubClassName=ps_input  LeftPortType=input  RightPortType=output  PseudoPeriodic=off  Frequencies=[]  NoiseDistribution=none  NoiseParameters=[]  Unit=1  AffineConversion=off  FilteringAndDerivatives=provide  SimscapeFilterOrder=1  InputFilterTimeConstant=0.001  UdotUserProvided=0
  Switch : Switch  Criteria=u2 > Threshold
  Voltage Sensor : fl_lib/Electrical/Electrical Sensors/Voltage Sensor
  Batt_+ : PMIOPort  Port=1  Side=Left
  " Batt_-" : PMIOPort  Port=2  Side=Left
  Out1 : Outport
  wires:
  Driver Signals/1 -> Input Signal Processing/3(Driver)
  Genset Inputs/1 -> Input Signal Processing/2(Genset)
  Component Cmds/1 -> Input Signal Processing/1(HSC Inputs)
  PS-Simulink Converter/1 -> [Batt_voltage_V]
  PS-Simulink Converter1/1 -> [Batt_current_A]
  Input Signal Processing/3(Aux Load) -> Product/1
  [Batt_voltage_V] -> Product/2
  Input Signal Processing/4(DC Mode) -> Switch/2
  Product/1 -> [gen_auxLoad_], Switch/1
  Constant/1 -> Switch/3
  [Batt_voltage_V] -> 2-D Lookup Table/2
  [Batt_current_A] -> 2-D Lookup Table/1
  2-D Lookup Table/1 -> Conditional Divide/2(u2)
  Switch/1 -> Conditional Divide/1(u1)
  Off/1 -> Conditional Divide/3(u3)
  Conditional Divide/1(Out1) -> Conditional Divide1/1(u1)
  [Batt_voltage_V] -> Conditional Divide1/2(u2)
  Off1/1 -> Conditional Divide1/3(u3)
  Off2/1 -> Conditional Divide2/3(u3)
  Input Signal Processing/2(gen_pwrElec_W) -> Gain/1
  [Batt_voltage_V] -> Conditional Divide2/2(u2)
  Gain/1 -> Conditional Divide2/1(u1)
  Conditional Divide2/1(Out1) -> Gain1/1
  Gain1/1 -> Add/1, [gen_gensetCurrent_A]
  Conditional Divide1/1(Out1) -> Add/2
  Add/1 -> Signal Processing/1(In1)
  Signal Processing/1(Out1) -> Simulink-PS Converter/1
  Input Signal Processing/1(gen_loadTrq_Nm) -> [gen_loadTrq_Nm]
  [Batt_current_A] -> Signal Porcessing/1(In1)
  [Batt_voltage_V] -> Signal Porcessing/2(In2)
  [gen_auxLoad_] -> Signal Porcessing/3(In3)
  [gen_gensetCurrent_A] -> Signal Porcessing/4(In4)
  [gen_loadTrq_Nm] -> Signal Porcessing/5(In5)
  Signal Porcessing/1(Out1) -> Out1/1
  connections:
  Current Sensor/LConn1 -- Batt_+/RConn1
  Controlled Current Source/LConn1 -- " Batt_-"/RConn1 -- Voltage Sensor/RConn2
  Current Sensor/RConn2 -- Voltage Sensor/LConn1 -- Controlled Current Source/RConn2
  Current Sensor/RConn1 -- PS-Simulink Converter1/LConn1
  Voltage Sensor/RConn1 -- PS-Simulink Converter/LConn1
  Simulink-PS Converter/RConn1 -- Controlled Current Source/RConn1

== system fullVehicleModel_17b/Vehicle Model/Variant Subsystem1/Subsystem1 ==
  Component Cmds : Inport
  Out1 : Outport

== system fullVehicleModel_17b/Vehicle Model/Variant Subsystem2/Subsystem ==
  In1 : Inport
  Out1 : Outport

== system fullVehicleModel_17b/Vehicle Model/Variant Subsystem2/Subsystem1 ==
  In1 : Inport
  Out1 : Outport

== system fullVehicleModel_17b/Controller Modules /Component Controllers/BMS Control Module/BMS Controller Module ==
  note: send help
  note: add all the conversion blocks
      | and name all the signals
  note: This is here becuase it is a feedback thing
  note: I have no idea what this is
  BMS_BMSEnable : Inport
  BMS_BMSEPO : Inport  Port=2
  BMS_mainContctClose : Inport  Port=3
  Batt_current_A : Inport  Port=4
  Batt_SOC_pct : Inport  Port=5
  Batt_temp_C : Inport  Port=6
  Batt_voltage_V : Inport  Port=7
  IgnitionCMD : Inport  Port=8
  BCM Constant Signals : Subsystem
  Bus Creator : BusCreator  Inputs=24
  EPO Check Enabler : Subsystem
  EPO_Check : Subsystem
  Memory1 : Memory  InheritSampleTime=on
  Startup Procedure : Stateflow chart  TreatAsAtomicUnit=on
  Subsystem : Subsystem
  Subsystem1 : Subsystem
  Unit Delay : UnitDelay  SampleTime=-1
  Unit Delay1 : UnitDelay  SampleTime=-1
  contactor logic : Subsystem
  Out1 : Outport
  Out2 : Outport  Port=2
  wires:
  Batt_current_A/1 -> Subsystem/1(Current), EPO Check Enabler/1(Current), Bus Creator/8
  Batt_temp_C/1 -> Bus Creator/10, EPO_Check/4(bat_temp), Subsystem/3(Temperature)
  Batt_SOC_pct/1 -> Subsystem/2(SOC), Bus Creator/9
  Subsystem/1(Chg_Buf_pct) -> Bus Creator/11, EPO Check Enabler/2(charge_buf)
  Subsystem/2(DisChg_Buf_pct) -> Bus Creator/12, EPO Check Enabler/3(discharge_buf)
  EPO Check Enabler/1(current_toEPO) -> EPO_Check/1(Current)
  Subsystem/3(Chg_max_A) -> Bus Creator/13, EPO_Check/2(Chg_max_amps)
  Subsystem/4(DisChg_max_A) -> Bus Creator/14, EPO_Check/3(DisChg_max_amps)
  BMS_mainContctClose/1 -> Unit Delay/1
  Unit Delay/1 -> Startup Procedure/1(hsc_bcm_mainc_close), contactor logic/2(contactor rqst)
  BMS_BMSEPO/1 -> contactor logic/1(hsc_epo)
  Startup Procedure/4(bcm_cpwr_cmd) -> contactor logic/3(contactor_pwr_cmd), Bus Creator/1
  contactor logic/2(contactor _status) -> Memory1/1
  BMS_BMSEnable/1 -> Unit Delay1/1
  Unit Delay1/1 -> Startup Procedure/4(hsc_bcm_enable)
  IgnitionCMD/1 -> Subsystem1/1(IgnitiionCMD)
  Subsystem1/1(Ignition) -> Startup Procedure/2(ignition)
  Subsystem1/2(ignition_status) -> Bus Creator/6, Startup Procedure/3(bcm_hvil_mon)
  EPO_Check/1(EPO_BCM) -> [EPO_BCM]
  [EPO_BCM] -> contactor logic/4(bcm_epo)
  Memory1/1 -> Bus Creator/5, Startup Procedure/5(bcm_mainc_stat)
  Startup Procedure/1(bcm_veh_mon) -> Bus Creator/2
  Startup Procedure/2(bcm_ready) -> Bus Creator/3
  Startup Procedure/3(bcm_cpwr_mon) -> Bus Creator/4
  Batt_voltage_V/1 -> Bus Creator/7
  Bus Creator/1 -> Out2/1
  contactor logic/1(contactor _signals) -> Out1/1
  [EPO_BCM] -> Bus Creator/15
  BCM Constant Signals/1(bcm_onPlug) -> Bus Creator/16
  BCM Constant Signals/2(bcm_alarm) -> Bus Creator/17
  BCM Constant Signals/3(bcm_gfd_kOhms) -> Bus Creator/18
  BCM Constant Signals/4(bcm_chgDone) -> Bus Creator/19
  BCM Constant Signals/5(bcm_coolReq) -> Bus Creator/20
  BCM Constant Signals/6(bcm_chgcStat) -> Bus Creator/21
  BCM Constant Signals/7(bcm_llsStatus) -> Bus Creator/22
  BCM Constant Signals/8(bcm_cellUndervolt) -> Bus Creator/23
  BCM Constant Signals/9(bcm_cellOvervolt) -> Bus Creator/24

== system fullVehicleModel_17b/Controller Modules /Component Controllers/BMS Control Module/Controller Inputs ==
  note: 1) Add Subsystem or Model blocks as valid variant choices.
      | 2) You cannot connect blocks at this level. At simulation, connectivity is automatically
      | determined, based on the active variant and port name matching.
  BattHSC : Inport
  BattPlant : Inport  Port=2
  IgnitionCMD : Inport  Port=3
  SiL Inputs : Subsystem  VariantControl=Variant
  BMS_BMSEnable : Outport
  BMS_BMSEPO : Outport  Port=2
  BMS_mainContctClose : Outport  Port=3
  Batt_current_A : Outport  Port=4
  Batt_SOC_pct : Outport  Port=5
  Batt_temp_C : Outport  Port=6
  Batt_voltage_V : Outport  Port=7
  IngnitionCMD : Outport  Port=8

== system fullVehicleModel_17b/Controller Modules /Component Controllers/BMS Control Module/Controller Outputs ==
  note: 1) Add Subsystem or Model blocks as valid variant choices.
      | 2) You cannot connect blocks at this level. At simulation, connectivity is automatically
      | determined, based on the active variant and port name matching.
  In1 : Inport
  In2 : Inport  Port=2
  SiL Controller Outputs : Subsystem  VariantControl=Variant
  Out1 : Outport
  Out2 : Outport  Port=2

== system fullVehicleModel_17b/Controller Modules /Component Controllers/Genset Control Module/Controller Inputs ==
  note: 1) Add Subsystem or Model blocks as valid variant choices.
      | 2) You cannot connect blocks at this level. At simulation, connectivity is automatically
      | determined, based on the active variant and port name matching.
  HSCCmd : Inport
  VehPlant : Inport  Port=2
  HiL Inputs : Subsystem  VariantControl=Variant1
  SiL Inputs : Subsystem  VariantControl=Variant
  eng_starterSwitchReq_bool : Outport
  Out2 : Outport  Port=2
  Out3 : Outport  Port=3
  Out4 : Outport  Port=4
  Out5 : Outport  Port=5
  Out6 : Outport  Port=6
  Out7 : Outport  Port=7
  Out8 : Outport  Port=8
  Out9 : Outport  Port=9
  Out10 : Outport  Port=10

== system fullVehicleModel_17b/Controller Modules /Component Controllers/Genset Control Module/Controller Outputs ==
  note: 1) Add Subsystem or Model blocks as valid variant choices.
      | 2) You cannot connect blocks at this level. At simulation, connectivity is automatically
      | determined, based on the active variant and port name matching.
  eng_enable : Inport
  eng_throttleReq_pct : Inport  Port=2
  gen_enable : Inport  Port=3
  gen_loadTrqReq_Nm : Inport  Port=4
  gen_pwrElec_kW : Inport  Port=5
  eng_engineSpd_rpm : Inport  Port=6
  eng_fuelLevelBit_bool : Inport  Port=7
  SiL Controller Outputs : Subsystem  VariantControl=Variant
  ToHSC : Outport
  PlantCmds : Outport  Port=2

== system fullVehicleModel_17b/Controller Modules /Component Controllers/Genset Control Module/Genset Controller Module ==
  In1 : Inport
  In2 : Inport  Port=2
  In3 : Inport  Port=3
  In4 : Inport  Port=4
  In5 : Inport  Port=5
  In6 : Inport  Port=6
  In7 : Inport  Port=7
  gen_pwrElec_kW : Inport  Port=8
  eng_engineSpd_rpm : Inport  Port=9
  eng_fuelLevelBit_bool : Inport  Port=10
  Engine Enable System : Subsystem
  Out1 : Outport
  Out2 : Outport  Port=2
  Out3 : Outport  Port=3
  Out4 : Outport  Port=4
  Out5 : Outport  Port=5
  Out6 : Outport  Port=6
  Out7 : Outport  Port=7
  wires:
  Engine Enable System/1(Out1) -> Out1/1  "enableSig"
  In2/1 -> Engine Enable System/2(In2)
  In3/1 -> Engine Enable System/3(In3)
  In6/1 -> Out3/1
  In1/1 -> Engine Enable System/1(In1)
  In4/1 -> Engine Enable System/4(In4)
  In7/1 -> Out4/1
  In5/1 -> Out2/1
  eng_fuelLevelBit_bool/1 -> Out7/1  "eng_fuelLevelBit_bool"
  eng_engineSpd_rpm/1 -> Out6/1
  gen_pwrElec_kW/1 -> Out5/1

== system fullVehicleModel_17b/Controller Modules /Component Controllers/INVCON Controller Module/Controller Inputs ==
  note: 1) Add Subsystem or Model blocks as valid variant choices.
      | 2) You cannot connect blocks at this level. At simulation, connectivity is automatically
      | determined, based on the active variant and port name matching.
  HSCCmd : Inport
  VehPlant : Inport  Port=2
  SiL Inputs : Subsystem  VariantControl=Variant
  HV_Dmd : Outport
  HV_CurrDmd : Outport  Port=2
  LV_CurrDmd : Outport  Port=3
  LV_Dmd : Outport  Port=4
  DCDC_ModeReq : Outport  Port=5
  HV_current : Outport  Port=6
  HV_volt : Outport  Port=7
  Aux_load : Outport  Port=8
  gen_GenCurrent_A : Outport  Port=9
  gen_loadTrq_Nm : Outport  Port=10

== system fullVehicleModel_17b/Controller Modules /Component Controllers/INVCON Controller Module/Controller Outputs ==
  note: 1) Add Subsystem or Model blocks as valid variant choices.
      | 2) You cannot connect blocks at this level. At simulation, connectivity is automatically
      | determined, based on the active variant and port name matching.
  HV_DCVoltage_V : Inport
  LV_DCCurrent_A : Inport  Port=2
  DC_Mode : Inport  Port=3
  HV_DCCurrent_A : Inport  Port=4
  DC_Temp : Inport  Port=5
  LV_DCVoltage_V : Inport  Port=6
  gen_GenCurrent_A : Inport  Port=7
  gen_loadTrq_Nm : Inport  Port=8
  SiL Controller Outputs : Subsystem  VariantControl=Variant
  INVToHSC : Outport

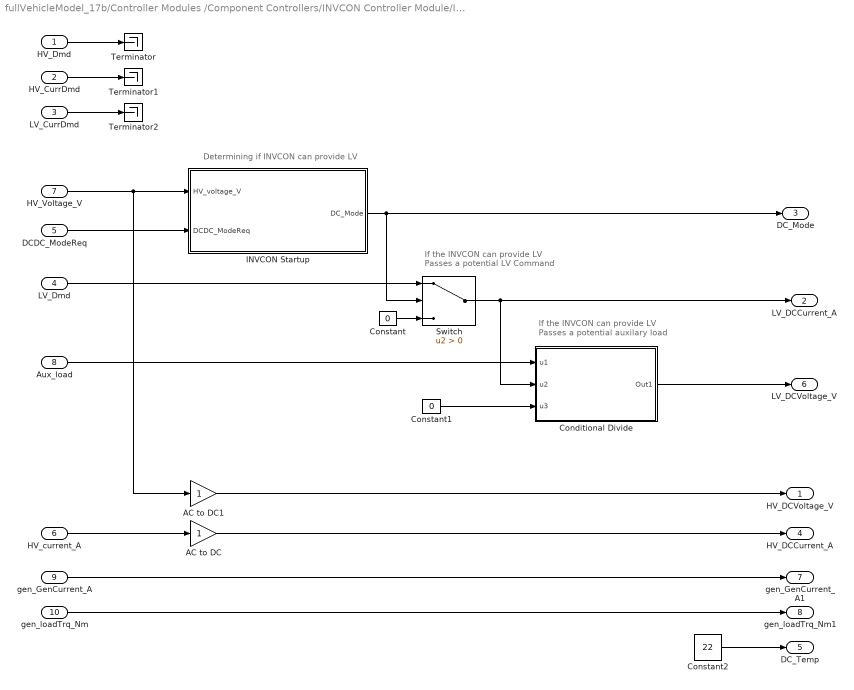
== system fullVehicleModel_17b/Controller Modules /Component Controllers/INVCON Controller Module/INVCON Controller Module ==
  note: If the INVCON can provide LV
      | Passes a potential LV Command
  note: Determining if INVCON can provide LV
  note: If the INVCON can provide LV
      | Passes a potential auxilary load
  HV_Dmd : Inport
  HV_CurrDmd : Inport  Port=2
  LV_CurrDmd : Inport  Port=3
  LV_Dmd : Inport  Port=4
  DCDC_ModeReq : Inport  Port=5
  HV_current_A : Inport  Port=6
  HV_Voltage_V : Inport  Port=7
  Aux_load : Inport  Port=8
  gen_GenCurrent_A : Inport  Port=9
  gen_loadTrq_Nm : Inport  Port=10
  AC to DC : Gain
  AC to DC1 : Gain
  Conditional Divide : Subsystem
  Constant : Constant  Value=0
  Constant1 : Constant  Value=0
  Constant2 : Constant  Value=22
  INVCON Startup : Stateflow chart  TreatAsAtomicUnit=on
  Switch : Switch  Criteria=u2 > Threshold
  Terminator : Terminator
  Terminator1 : Terminator
  Terminator2 : Terminator
  HV_DCVoltage_V : Outport
  LV_DCCurrent_A : Outport  Port=2
  DC_Mode : Outport  Port=3
  HV_DCCurrent_A : Outport  Port=4
  DC_Temp : Outport  Port=5
  LV_DCVoltage_V : Outport  Port=6
  gen_GenCurrent_A1 : Outport  Port=7
  gen_loadTrq_Nm1 : Outport  Port=8
  wires:
  HV_Voltage_V/1 -> INVCON Startup/1(HV_voltage_V), AC to DC1/1
  DCDC_ModeReq/1 -> INVCON Startup/2(DCDC_ModeReq)
  LV_Dmd/1 -> Switch/1
  Constant/1 -> Switch/3
  Aux_load/1 -> Conditional Divide/1(u1)
  INVCON Startup/1(DC_Mode) -> Switch/2, DC_Mode/1
  Constant1/1 -> Conditional Divide/3(u3)
  Switch/1 -> Conditional Divide/2(u2), LV_DCCurrent_A/1
  Conditional Divide/1(Out1) -> LV_DCVoltage_V/1
  HV_current_A/1 -> AC to DC/1
  AC to DC/1 -> HV_DCCurrent_A/1
  AC to DC1/1 -> HV_DCVoltage_V/1
  gen_GenCurrent_A/1 -> gen_GenCurrent_A1/1
  gen_loadTrq_Nm/1 -> gen_loadTrq_Nm1/1
  Constant2/1 -> DC_Temp/1
  HV_Dmd/1 -> Terminator/1
  HV_CurrDmd/1 -> Terminator1/1
  LV_CurrDmd/1 -> Terminator2/1
